simulink model "addLastKeyEventRefMod"  (R2016b)
settings: Solver=VariableStepAuto  StartTime=0.0  StopTime=10.0  RelTol=1e-3
settings Model: DataDictionary=DataDictionary.sldd  Creator=Taeke  LastModifiedBy=Nathan
settings DataIOCC: SaveOutput=off

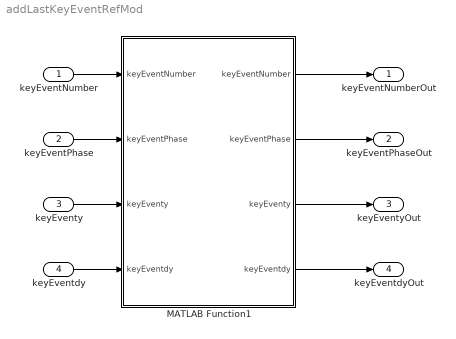
== system addLastKeyEventRefMod ==
  keyEventNumber : Inport
  keyEventPhase : Inport  Port=2  PortDimensions=keyEventsAmount
  keyEventy : Inport  Port=3  PortDimensions=keyEventsAmount
  keyEventdy : Inport  Port=4  PortDimensions=keyEventsAmount
  MATLAB Function1 : MATLAB Function  TreatAsAtomicUnit=on
  keyEventNumberOut : Outport
  keyEventPhaseOut : Outport  Port=2
  keyEventyOut : Outport  Port=3
  keyEventdyOut : Outport  Port=4
  wires:
  keyEventNumber/1 -> MATLAB Function1/1("keyEventNumber ")
  keyEventPhase/1 -> MATLAB Function1/2("keyEventPhase ")
  keyEventy/1 -> MATLAB Function1/3("keyEventy ")
  keyEventdy/1 -> MATLAB Function1/4("keyEventdy ")
  MATLAB Function1/1(keyEventNumber) -> keyEventNumberOut/1
  MATLAB Function1/2(keyEventPhase) -> keyEventPhaseOut/1
  MATLAB Function1/3(keyEventy) -> keyEventyOut/1
  MATLAB Function1/4(keyEventdy) -> keyEventdyOut/1

== matlab function addLastKeyEventRefMod/MATLAB Function1 ==
  data: keyEventNumber input; keyEventNumber output; keyEventPhase input; keyEventy input; keyEventdy input; keyEventPhase output; keyEventy output; keyEventdy output
function [keyEventNumber, keyEventPhase,keyEventy,keyEventdy] = addLastKeyEvent(keyEventNumber, keyEventPhase,keyEventy,keyEventdy)
[keyEventNumber, keyEventPhase,keyEventy,keyEventdy] = add_last_key_event(keyEventNumber, keyEventPhase,keyEventy,keyEventdy);
